simulink model "Module_Simulation"  (R2017b)
settings: Solver=FixedStepAuto  StartTime=0.0  StopTime=1000000  FixedStep=0.1  MaxStep=1e-4  RelTol=1e-3
values from neighbouring files (symbols this model uses):
  Capacity_max = 3113 * N_Cell    (= 3113)    [Battery_Parameters.m]    (also in Module_Spec.m = zeros(1,Nb_cell_module); SOC_Curve.m = SOC_data(end,1); Test_spec.m = Capacity_max_norm3)
  I_discharge = C_mean    [Test_spec.m]
  R0 = 0.0715 / N_Cell    (= 0.0715)    [Battery_Parameters.m]    (also in Module_Spec.m = zeros(1,Nb_cell_module); Test_spec.m = R0_norm1)
undefined symbols (not defined in the file or in its folder): Ion, Lithium
libraries: electricdrivelib x6, powerlib x2, simulink x1
settings Model: Creator=christian  LastModifiedBy=christian

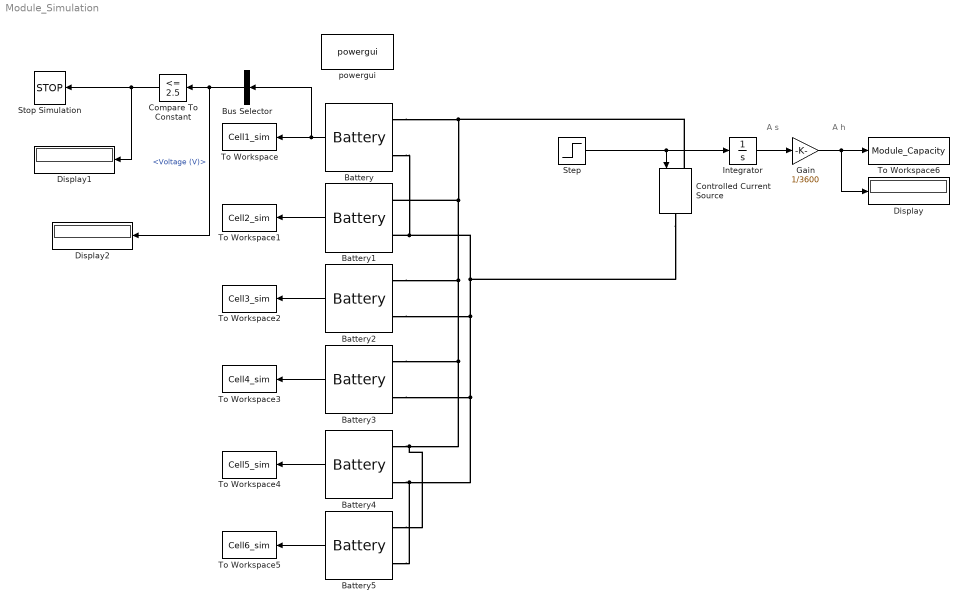
== system Module_Simulation ==
  note: A s
  note: A h
  Battery : electricdrivelib/Extra Sources/Battery  BatType=Lithium-Ion  ShowTempParam=off  ThermalPreset=no  ShowAgeParam=off  NomV=3.6  NomQ=Capacity_max(1)/1000  SOC=initial_SOC  Batt_Tr=100  PresetModel=off  MaxQ=Capacity_max(1)/1000  MinV=2.7  FullV=4.1904  Dis_rate=1  R=R0(1)  Normal_OP=Capacity_max(1)/1200  expZone="[3.8894    0.08*Capacity_max(1)/1000]"  current=[1]  Units=Ampere-hour  Tci=20  NomT=20  T2=-30  MaxQ2=4.8  FullV2=7.1  Normal_OP2=5.655  expZone2="[6.58           1]"  Rca=0.6  ti=2000  Dp=0  Neq0=0  Tsim=1e6  Ta1=25  Qeol=5.4*0.9  Reol=0.013333*1.2  Char_age=[2.3478, 3]  Dis_age=[2.3478, 10]  N1=1500  N2=10500  N3=1000  N4=1400  Ta2=45  N5=950
  Battery1 : electricdrivelib/Extra Sources/Battery  BatType=Lithium-Ion  ShowTempParam=off  ThermalPreset=no  ShowAgeParam=off  NomV=3.6  NomQ=Capacity_max(2)/1000  SOC=initial_SOC  Batt_Tr=100  PresetModel=off  MaxQ=Capacity_max(2)/1000  MinV=2.5  FullV=4.2  Dis_rate=1  R=R0(2)*1e-3  Normal_OP=Capacity_max(2)/1200  expZone="[3.92     0.08*Capacity_max(2)/1000]"  current=[1]  Units=Ampere-hour  Tci=20  NomT=20  T2=-30  MaxQ2=4.8  FullV2=7.1  Normal_OP2=5.655  expZone2="[6.58           1]"  Rca=0.6  ti=2000  Dp=0  Neq0=0  Tsim=1e6  Ta1=25  Qeol=5.4*0.9  Reol=0.013333*1.2  Char_age=[2.3478, 3]  Dis_age=[2.3478, 10]  N1=1500  N2=10500  N3=1000  N4=1400  Ta2=45  N5=950
  Battery2 : electricdrivelib/Extra Sources/Battery  BatType=Lithium-Ion  ShowTempParam=off  ThermalPreset=no  ShowAgeParam=off  NomV=3.6  NomQ=Capacity_max(3)/1000  SOC=initial_SOC  Batt_Tr=100  PresetModel=off  MaxQ=Capacity_max(3)/1000  MinV=2.5  FullV=4.2  Dis_rate=1  R=R0(3)*1e-3  Normal_OP=Capacity_max(3)/1200  expZone="[3.92     0.08*Capacity_max(3)/1000]"  current=[1]  Units=Ampere-hour  Tci=20  NomT=20  T2=-30  MaxQ2=4.8  FullV2=7.1  Normal_OP2=5.655  expZone2="[6.58           1]"  Rca=0.6  ti=2000  Dp=0  Neq0=0  Tsim=1e6  Ta1=25  Qeol=5.4*0.9  Reol=0.013333*1.2  Char_age=[2.3478, 3]  Dis_age=[2.3478, 10]  N1=1500  N2=10500  N3=1000  N4=1400  Ta2=45  N5=950
  Battery3 : electricdrivelib/Extra Sources/Battery  BatType=Lithium-Ion  ShowTempParam=off  ThermalPreset=no  ShowAgeParam=off  NomV=3.6  NomQ=Capacity_max(4)/1000  SOC=initial_SOC  Batt_Tr=100  PresetModel=off  MaxQ=Capacity_max(4)/1000  MinV=2.5  FullV=4.2  Dis_rate=1  R=R0(4)*1e-3  Normal_OP=Capacity_max(4)/1200  expZone="[3.92     0.08*Capacity_max(4)/1000]"  current=[1]  Units=Ampere-hour  Tci=20  NomT=20  T2=-30  MaxQ2=4.8  FullV2=7.1  Normal_OP2=5.655  expZone2="[6.58           1]"  Rca=0.6  ti=2000  Dp=0  Neq0=0  Tsim=1e6  Ta1=25  Qeol=5.4*0.9  Reol=0.013333*1.2  Char_age=[2.3478, 3]  Dis_age=[2.3478, 10]  N1=1500  N2=10500  N3=1000  N4=1400  Ta2=45  N5=950
  Battery4 : electricdrivelib/Extra Sources/Battery  BatType=Lithium-Ion  ShowTempParam=off  ThermalPreset=no  ShowAgeParam=off  NomV=3.6  NomQ=Capacity_max(5)/1000  SOC=initial_SOC  Batt_Tr=100  PresetModel=off  MaxQ=Capacity_max(5)/1000  MinV=2.5  FullV=4.2  Dis_rate=1  R=R0(5)*1e-3  Normal_OP=Capacity_max(5)/1200  expZone="[3.92     0.08*Capacity_max(5)/1000]"  current=[1]  Units=Ampere-hour  Tci=20  NomT=20  T2=-30  MaxQ2=4.8  FullV2=7.1  Normal_OP2=5.655  expZone2="[6.58           1]"  Rca=0.6  ti=2000  Dp=0  Neq0=0  Tsim=1e6  Ta1=25  Qeol=5.4*0.9  Reol=0.013333*1.2  Char_age=[2.3478, 3]  Dis_age=[2.3478, 10]  N1=1500  N2=10500  N3=1000  N4=1400  Ta2=45  N5=950
  Battery5 : electricdrivelib/Extra Sources/Battery  BatType=Lithium-Ion  ShowTempParam=off  ThermalPreset=no  ShowAgeParam=off  NomV=3.6  NomQ=Capacity_max(6)/1000  SOC=initial_SOC  Batt_Tr=100  PresetModel=off  MaxQ=Capacity_max(6)/1000  MinV=2.5  FullV=4.2  Dis_rate=1  R=R0(6)*1e-3  Normal_OP=Capacity_max(6)/1200  expZone="[3.92     0.08*Capacity_max(6)/1000]"  current=[1]  Units=Ampere-hour  Tci=20  NomT=20  T2=-30  MaxQ2=4.8  FullV2=7.1  Normal_OP2=5.655  expZone2="[6.58           1]"  Rca=0.6  ti=2000  Dp=0  Neq0=0  Tsim=1e6  Ta1=25  Qeol=5.4*0.9  Reol=0.013333*1.2  Char_age=[2.3478, 3]  Dis_age=[2.3478, 10]  N1=1500  N2=10500  N3=1000  N4=1400  Ta2=45  N5=950
  Bus Selector : BusSelector  OutputSignals=Voltage (V)
  Compare To Constant : simulink/Logic and Bit Operations/Compare To Constant  relop=<=  const=2.5  OutDataTypeStr=boolean
  Controlled Current Source : powerlib/Electrical Sources/Controlled Current Source  Initialize=on  Source_Type=DC  Amplitude=0  Phase=0  Frequency=0  Measurements=None
  Display : Display
  Display1 : Display
  Display2 : Display
  Gain : Gain  Gain=1/3600
  Integrator : Integrator
  Step : Step  After=I_discharge/1000  SampleTime=0
  Stop Simulation : Stop
  To Workspace : ToWorkspace  VariableName=Cell1_sim  SaveFormat=Timeseries  SampleTime=-1
  To Workspace1 : ToWorkspace  VariableName=Cell2_sim  SaveFormat=Timeseries  SampleTime=-1
  To Workspace2 : ToWorkspace  VariableName=Cell3_sim  SaveFormat=Timeseries  SampleTime=-1
  To Workspace3 : ToWorkspace  VariableName=Cell4_sim  SaveFormat=Timeseries  SampleTime=-1
  To Workspace4 : ToWorkspace  VariableName=Cell5_sim  SaveFormat=Timeseries  SampleTime=-1
  To Workspace5 : ToWorkspace  VariableName=Cell6_sim  SaveFormat=Timeseries  SampleTime=-1
  To Workspace6 : ToWorkspace  VariableName=Module_Capacity  SaveFormat=Timeseries  SampleTime=-1
  powergui : powerlib/powergui  Priority=1  SimulationMode=Discrete  SampleTime=0.1  frequency=60  Iterations=50  frequencyindice=0  Pbase=100e6  ErrMax=1e-4  UnitsV=kV  UnitsW=MW  buscounter=0  FunctionMessages=off  echomessages=off  EnableUseOfTLC=off  CurrentSourceSwitches=off  DisableSnubberDevices=off  DisableRonSwitches=off  DisableVfSwitches=off  DisplayEquations=off  SolverType=Tustin/Backward Euler (TBE)  Interpol=off  ExternalGateDelay=off  methode=off  Ts=100  x0status=blocks  SPID=off  SwTol=0  HookPort=off  RestoreLinks=warning  ResistiveCurrentMeasurement=off  Frange=[0:2:500]  Ylog=off  Xlog=on  ShowGrid=off  save=off  variable=ZData  structure=0  ZoomFFT=off  StartTime=0.0  cycles=1  DisplayStyle=1  fundamental=60  FreqAxis=off  MaxFrequency=1000  frequencyindicesteady=1  RmsSteady=1  display=off
  wires:
  Battery/1 -> Bus Selector/1, To Workspace/1
  Battery1/1 -> To Workspace1/1
  Step/1 -> Integrator/1, Controlled Current Source/1
  Battery2/1 -> To Workspace2/1
  Battery3/1 -> To Workspace3/1
  Battery4/1 -> To Workspace4/1
  Battery5/1 -> To Workspace5/1
  Integrator/1 -> Gain/1
  Gain/1 -> Display/1, To Workspace6/1
  Bus Selector/1 -> Display2/1, Compare To Constant/1  "<Voltage (V)>"
  Compare To Constant/1 -> Display1/1, Stop Simulation/1
  connections:
  Battery/LConn1 -- Controlled Current Source/LConn1 -- Battery2/LConn1 -- Battery3/LConn1 -- Battery5/LConn1 -- Battery4/LConn1 -- Battery1/LConn1
  Battery/LConn2 -- Battery1/LConn2 -- Battery2/LConn2 -- Battery3/LConn2 -- Battery5/LConn2 -- Battery4/LConn2 -- Controlled Current Source/RConn1
